simulink model "SystemWithConversionsComponent"  (R2017b)
settings: Solver=ode8  StartTime=0.0  StopTime=5  FixedStep=0.01  RelTol=1e-3
InitFcn:
  | ra = 4;
  | jm = 0.0000218;
  | rm = 0.7/100;
  | dsm = 62.892;
  | kt = 0.138;
  | ke = kt;
  | ms = 0.93;
  | hl = 1.5 / 100;
  | Lr = 24.1 / 100;
  | Lcm = hl / 2 + Lr;
  | ml =0.182;
  | mr = 0.085;
  | rl = 20.125 / 1000;
  | Jp =1/3 * mr * Lr^2 + 1/2*ml*rl^2 + ml * Lcm ^ 2;
  | Dp = 0.007;
  | g = 9.82;
StartFcn:
  | ra = 4;
  | jm = 0.0000218;
  | rm = 0.7/100;
  | dsm = 62.892;
  | kt = 0.138;
  | ke = kt;
  | ms = 0.93;
undefined symbols (not defined in the file or in its folder): National_Instruments, PCI
libraries: sldrtlib x4
settings Model: Creator=labadmin  LastModifiedBy=labadmin
settings DataIOCC: SaveOutput=off  SaveTime=off
settings RTWCC: SystemTargetFile=sldrt.tlc  TemplateMakefile=sldrt.tmf  Description=Simulink Desktop Real-Time  RTWCompilerOptimization=on
settings CodeAppCC: MaxIdLength=95
settings SimulinkDesktopRealTimeCC: TargetPreCompLibLocation=C:\Program Files\MATLAB\R2017b\toolbox\sldrt\lib\win64

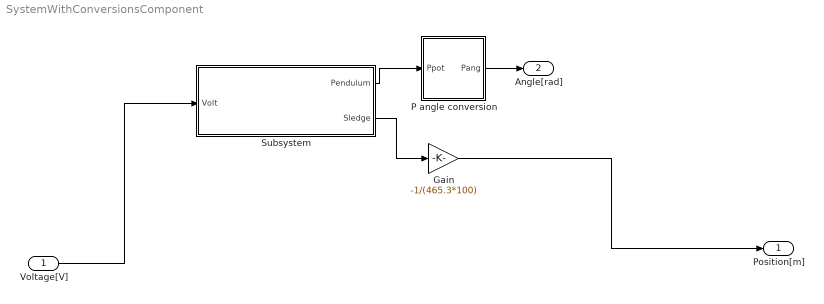
== system SystemWithConversionsComponent ==
  Voltage[V] : Inport  OutDataTypeStr=double  PortDimensions=1  SampleTime=0
  Gain : Gain  Gain=-1/(465.3*100)
  P angle conversion : Subsystem
  Subsystem : Subsystem
  Position[m] : Outport  OutDataTypeStr=double  PortDimensions=1  SampleTime=[0.01,0]
  Angle[rad] : Outport  Port=2  OutDataTypeStr=double  PortDimensions=1  SampleTime=[0.01,0]
  wires:
  Gain/1 -> Position[m]/1
  P angle conversion/1(Pang) -> Angle[rad]/1
  Subsystem/2(Sledge) -> Gain/1
  Subsystem/1(Pendulum) -> P angle conversion/1(Ppot)
  Voltage[V]/1 -> Subsystem/1(Volt)

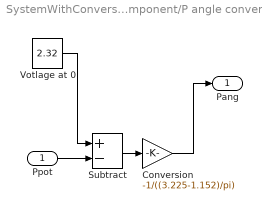
== system SystemWithConversionsComponent/P angle conversion ==
  Ppot : Inport
  Conversion : Gain  Gain=-1/((3.225-1.152)/pi)
  Subtract : Sum  Inputs=+-
  "Votlage at 0 " : Constant  Value=2.32
  Pang : Outport
  wires:
  Conversion/1 -> Pang/1
  "Votlage at 0 "/1 -> Subtract/1
  Ppot/1 -> Subtract/2
  Subtract/1 -> Conversion/1

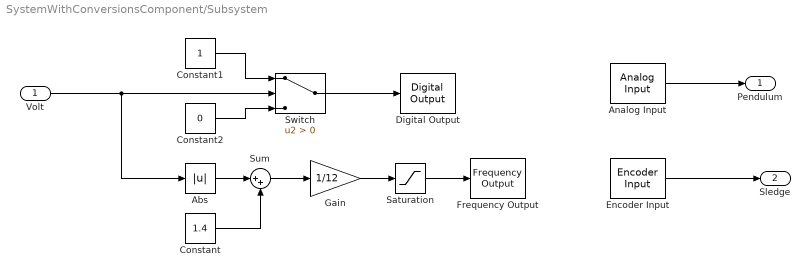
== system SystemWithConversionsComponent/Subsystem ==
  Volt : Inport
  Abs : Abs
  Analog Input : sldrtlib/Analog Input  SampleTime=-1  MaxMissedTicks=1000000000  ShowMissedTicks=off  YieldWhenWaiting=off  DrvName=National_Instruments/PCI-6229  DrvAddress=4294967295  DrvOptions=[0 1 8192 2 3]  Channels=1  RangeMode=1  VoltRange=1  DataType=1
      settings: AttributesFormatString=National Instruments\nPCI-6229 [auto]  SourceProductName=Simulink Desktop Real-Time
  Constant : Constant  Value=1.4
  Constant1 : Constant
  Constant2 : Constant  Value=0
  Digital Output : sldrtlib/Digital Output  SampleTime=-1  MaxMissedTicks=100000000  ShowMissedTicks=off  YieldWhenWaiting=off  DrvName=National_Instruments/PCI-6229  DrvAddress=4294967295  DrvOptions=[0 1 8192 2 3]  Channels=1  BitMode=1  InitialValue=[]  FinalValue=[]
      settings: AttributesFormatString=National Instruments\nPCI-6229 [auto]  SourceProductName=Simulink Desktop Real-Time  SourceProductBaseCode=WT
  Encoder Input : sldrtlib/Encoder Input  SampleTime=-1  MaxMissedTicks=10000000  ShowMissedTicks=off  YieldWhenWaiting=off  DrvName=National_Instruments/PCI-6229  DrvAddress=4294967295  DrvOptions=[0 1 8192 2 3]  Channels=1  QuadMode=3  IndexPulse=2  InputFilter=Inf  DataType=1
      settings: AttributesFormatString=National Instruments\nPCI-6229 [auto]  SourceProductName=Simulink Desktop Real-Time
  Frequency Output : sldrtlib/Frequency Output  SampleTime=-1  MaxMissedTicks=1000000000  ShowMissedTicks=off  YieldWhenWaiting=off  DrvName=National_Instruments/PCI-6229  DrvAddress=4294967295  DrvOptions=[0 1 8192 2 3]  Channels=2  FrequencySource=1  Frequency=10000  FrequencyFinalValue=[]  DutySource=2  Duty=0  DutyFinalValue=0
      settings: AttributesFormatString=National Instruments\nPCI-6229 [auto]  SourceProductName=Simulink Desktop Real-Time  SourceProductBaseCode=WT
  Gain : Gain  Gain=1/12
  Saturation : Saturate  LowerLimit=0
  Sum : Sum  Inputs=|++
  Switch : Switch  Criteria=u2 > Threshold
  Pendulum : Outport
  Sledge : Outport  Port=2
  wires:
  Constant/1 -> Sum/2
  Sum/1 -> Gain/1
  Abs/1 -> Sum/1
  Switch/1 -> Digital Output/1
  Constant1/1 -> Switch/1
  Constant2/1 -> Switch/3
  Gain/1 -> Saturation/1
  Volt/1 -> Switch/2, Abs/1
  Saturation/1 -> Frequency Output/1
  Encoder Input/1 -> Sledge/1
  Analog Input/1 -> Pendulum/1
